simulink subsystem "TorqueControl"  (R2022a)
settings: Solver=VariableStepAuto  StartTime=0.0  StopTime=10.0  RelTol=1e-3
undefined symbols (not defined in the file): R, VS_Rgn2K_Nmprad2ps2
settings Model: Creator=jhummel  LastModifiedBy=jhummel

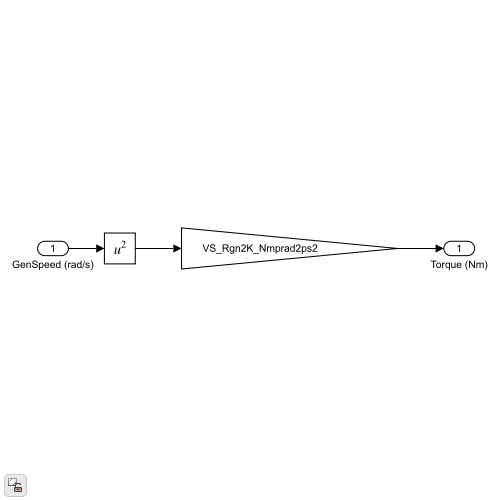
[thumbnail: Simulink's stored preview of the top-level diagram]
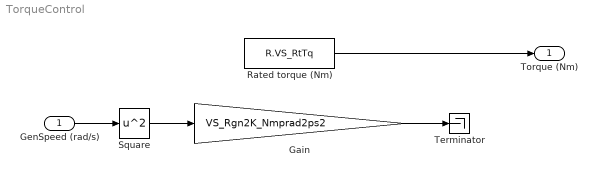
== system TorqueControl ==
  GenSpeed (rad/s) : Inport
  Gain : Gain  Gain=VS_Rgn2K_Nmprad2ps2
  Rated torque (Nm) : Constant  Value=R.VS_RtTq
  Square : Math  Operator=square
  Terminator : Terminator
  Torque (Nm) : Outport
  wires:
  GenSpeed (rad/s)/1 -> Square/1
  Square/1 -> Gain/1
  Rated torque (Nm)/1 -> Torque (Nm)/1
  Gain/1 -> Terminator/1
